simulink library "lib_Conduction_2DCondFullyImplicit"  (R2015a)
settings: Solver=ode45  StartTime=0.0  StopTime=10.0  RelTol=1e-3
libraries: lib_GenTools_SubMatrix x24
(part 2 of 2)

== matlab function lib_Conduction_2DCondFullyImplicit/2D Transient Conduction Model - Fully Implicit/MATLAB Function ==
  data: kx input; ky input; T output; Cp input; rho input; TfL input; hL input; TsL input; CL input; TrL input; uL input; TfR input; hR input; TsR input; CR input; TrR input; uR input; TfB input; hB input; TsB input; CB input; TrB input; uB input; TfT input; hT input; TsT input; CT input; TrT input; uT input; x input; y input; shape input; AL input; AR input; AB input; AT input; VL input; VR input; VB input; VT input; JLx input; JLy input; JRx input; JRy input; JBx input; JBy input; JTx input; JTy input; dt input; To input; Erro input; Err output; BN input
function [T,Err] = HeatX2DQuasi(kx,ky,Cp,rho,TfL,hL,...
    TsL,CL,TrL,uL,TfR,hR,TsR,CR,...
    TrR,uR,TfB,hB,TsB,CB,TrB,uB,TfT,hT,...
    TsT,CT,TrT,uT,x,y,shape,...
    AL,AR,AB,AT,VL,VR,VB,VT,JLx,JLy,JRx,JRy,...
    JBx,JBy,JTx,JTy,dt,To,Erro,BN)
%#codegen

% Written by: Jonathan Kratz, NASA GRC
% Date: January 27, 2017
%
% Description: This MATLAB function block solves a 2-D heat transfer
% problem with the potential for various boundary conditions including
% convection, conduction, and radiation. The function is capable of
% accepting time-varying thermal properties including the conductivity,
% specific heat, and density of the solid structure. Heat transfer
% coefficients can also be time-varying. The function is equiped to handle
% planar and cylindrical geometries. A generic non-uniform spatial
% discretization may be used but a constant time-step is encouraged for
% accuracy in time. The governing equation is below:
%                  _                                                  _
%   dT     1      |  /dk   a*k \ dT     d2T    /dk   q*k \  dT     d2T |
%   -- = ------ * | | -- + ---- |-- + k --- + | -- + ---- | -- + k --- |
%   dt   rho*Cp   |_ \dy    dy / dy     dy2    \dx    dx /  dx     dx2_|
%
% Generally the geometry will be planar in the x or y direction but could be
% axisymmetric (cylindrical) in the other direction. This equation is
% discretized and to form a system of linear equations and solved using a 2-D
% implicit scheme. The Crank-Nicolson Method is applied to the discretizied 
% equation and the linear algreba techniques are used to solve the system of 
% equations. The boundary conditions use linear heat transfer 
% coefficients and it is suggested that these coefficients be evaluated 
% using thermal properties of the previous time-step (i.e. temperature of 
% the structure and thermodynamic properties of the surrounding gases).
% Depending on the problem they may be assumed constant.
%
% Inputs:
%   Note m is the number of nodes in y-dir and n is the number of
%   nodes in the x-dir.
% Thermal Properties:
%   kx - thermal conductivity of the structure in x-dir [m x n]
%   ky - thermal conductivity of the structure in y-dir [m x n]
%   Cp - heat capacity of the structure [m x n]
%   rho - density of the structure [m x n]
% Boundary Conditions:
%   TfL - temperature of fluid on the left surface [m x 1]
%   hL - convective heat transfer coefficient on the left surface [m x 1]
%   CL - thermal conductance of contacting structure on the left surface 
%        [m x 1]
%   TsL - temperature of a contacting structure on the left surface [m x 1]
%   TrL - temperature of a distant external radiating source/sink [m x 1]
%       exposed to the left surface
%   uL - linear radiative heat transfer coefficient between the left
%       surface and external radiating source/sink it is exposed to [m x 1]
%   TfR - temperature of fluid on the right surface [m x 1]
%   hR - convective heat transfer coefficient on the right surface [m x 1]
%   TsR - temperature of a contacting structure on the right surface [m x 1]
%   CR - thermal conductance of contacting structure on the right surface 
%        [m x 1]
%   TrR - temperature of a distant external radiating source/sink
%       exposed to the right surface [m x 1]
%   uR - linear radiative heat transfer coefficient between the right
%       surface and external radiating source/sink it is exposed to [m x 1]
%   TfB - temperature of fluid on the bottom surface [n x 1]
%   hB - convective heat transfer coefficient on the bottom surface [n x 1]
%   TsB - temperature of a contacting structure on the bottom surface [n x 1]
%   CB - thermal conductance of contacting structure on the bottom surface 
%        [n x 1]
%   TrB - temperature of a distant external radiating source/sink 
%       exposed to the bottom surface [n x 1]
%   uB - linear radiative heat transfer coefficient between the bottom
%       surface and external radiating source/sink it is exposed to [n x 1]
%   TfT - temperature of fluid on the top surface [n x 1]
%   hT - convective heat transfer coefficient on the top surface [n x 1]
%   TsT - temperature of a contacting structure on the top surface [n x 1]
%   CT - thermal conductance of contacting structure on the top surface 
%        [n x 1]
%   TrT - temperature of a distant external radiating source/sink 
%       exposed to the top surface [n x 1]
%   uT - linear radiative heat transfer coefficient between the top
%       surface and external radiating source/sink it is exposed to [n x 1]
% Boundary Node Properties
%   AL - surface area of the left surface nodes [m x 1]
%   AR - surface area of the right surface nodes [m x 1]
%   AB - surface area of the bottom surface nodes [n x 1]
%   AT - surface area of the top surface nodes [n x 1]
%   VL - volume of the left surface nodes [m x 1]
%   VR - volume of the right surface nodes [m x 1]
%   VB - volume of the bottom surface nodes [n x 1]
%   VT - volume of the top surface nodes [n x 1]
%   JL - thermal resistance * k of the left surface nodes [m x 1]
%   JR - thermal resistance * k of the right surface nodes [m x 1]
%   JB - thermal resistance * k of the bottom surface nodes [n x 1]
%   JT - thermal resistance * k of the top surface nodes [n x 1]
% Geometry/Discretization:
%   x - discretized spatial coordinates in x-direction [n]
%   y - discretized spatial coordinates in r- or y-direction [m]
%   shape - shape parameter 
% Solver:
%   dt - time-step of the solver [1 x 1]
%   To - initial/previous condition for the solver/initial temperature of 
%       the structure [m x n]
% Error/Warning Detection
%   Erro - array with error states. Tracks errors/warnings that have been
%       detected. [number of error checks x 1]
%   BN - block name. Used in warning messages.
%
% Outputs:
%   T - Matrix of temperature at each node [m x n]
%   Err - array with updated error states. [number of error checks x 1]
%  
% Discretization guidelines: The first and last nodes should be on the 
% surface. It is important that that the first node should be half the size 
% as the second node and the last node should be half the size of the 
% second to last node. This is due to the assumptions made in the 
% formulization of the boundary condition equations. Also, for planar 
% geometries the first value of the discretization array x (which 
% corresponds to the first node) can be any real numeric value (it does not
% have to be zero, equations use node size so relative position is what 
% matters). In the case of a cylindrical geometry the first value in the x 
% array should be the inner radius of the structure. It should go without 
% saying that the spatial discretization array x is required to be 
% montonically increasing.

% shape factor
a = 0;
q = 0;
if shape == 1
    a = 0;
    q = 0;
elseif shape == 2
    a = 1;
    q = 0;
elseif shape == 3
    a = 0;
    q = 1;
end

% number of elements
n = length(x); %number of nodes in x-dir
m = length(y); %number of nodes in y-dir

% initialize error/warning array
Err = Erro;
ErrNum = 1; %Error index

%180 Error Checks
% check sizes and contents -----------------------------------------------%
% ---- x ---- %
% Not Empty?
if isempty(x) == 1 && Err(ErrNum) < 1
    Err(ErrNum) = 1;
    fprintf('Warning in %s: x_M is an empty array.\n',char(BN));
end
ErrNum = ErrNum + 1;
% 1-D Array?
if (length(size(x)) ~= 2 && min(size(x)) ~= 1) && Err(ErrNum) < 1
    Err(ErrNum) = 1;
    fprintf('Warning in %s: x_M must be a 1-D array.\n',char(BN));
end
ErrNum = ErrNum + 1;
% Length >= 4?
if length(x) < 4 && Err(ErrNum) < 1
    Err(ErrNum) = 1;
    fprintf('Warning in %s: x_M must have at least 4 elements.\n',char(BN));
end
ErrNum = ErrNum + 1;
% Real?
if min(isreal(x)) < 1 && Err(ErrNum) < 1
    Err(ErrNum) = 1;
    fprintf('Warning in %s: x_M must have all real elements.\n',char(BN));
end
ErrNum = ErrNum + 1;
% Finite?
if min(isfinite(x)) < 1 && Err(ErrNum) < 1
    Err(ErrNum) = 1;
    fprintf('Warning in %s: x_M must have all finite elements.\n',char(BN));
end
ErrNum = ErrNum + 1;
% Monotonically Increasing?
if min(diff(x)) <= 0 && Err(ErrNum) < 1
    Err(ErrNum) = 1;
    fprintf('Warning in %s: x_M must be monotonically increasing.\n',char(BN));
end
ErrNum = ErrNum + 1;
% ---- y ---- %
% Not Empty?
if isempty(y) == 1 && Err(ErrNum) < 1
    Err(ErrNum) = 1;
    fprintf('Warning in %s: y_M is an empty array.\n',char(BN));
end
ErrNum = ErrNum + 1;
% 1-D Array?
if (length(size(y)) ~= 2 && min(size(y)) ~= 1) && Err(ErrNum) < 1
    Err(ErrNum) = 1;
    fprintf('Warning in %s: y_M must be a 2-D array.\n',char(BN));
end
ErrNum = ErrNum + 1;
% Number of rows >= 4?
if length(y) < 4 && Err(ErrNum) < 1
    Err(ErrNum) = 1;
    fprintf('Warning in %s: y_M must have at least 4 rows.\n',char(BN));
end
ErrNum = ErrNum + 1;
% Real?
if min(isreal(y)) < 1 && Err(ErrNum) < 1
    Err(ErrNum) = 1;
    fprintf('Warning in %s: y_M must have all real elements.\n',char(BN));
end
ErrNum = ErrNum + 1;
% Finite?
if min(isfinite(y)) < 1 && Err(ErrNum) < 1
    Err(ErrNum) = 1;
    fprintf('Warning in %s: y_M must have all finite elements.\n',char(BN));
end
ErrNum = ErrNum + 1;
% y is Monotonically Increasing?
if min(diff(y)) <= 0 && Err(ErrNum) < 1
    Err(ErrNum) = 1;
    fprintf('Warning in %s: y_M must be monotonically increasing.\n',char(BN));
end
ErrNum = ErrNum + 1;
% ---- kx ---- %
% Not Empty?
if isempty(kx) == 1 && Err(ErrNum) < 1
    Err(ErrNum) = 1;
    fprintf('Warning in %s: kx is an empty array.\n',char(BN));
end
ErrNum = ErrNum + 1;
% Size of To?
if (size(kx,1) ~= m && size(kx,2) ~= n) && Err(ErrNum) < 1
    Err(ErrNum) = 1;
    fprintf('Warning in %s: kx must have as many rows a elements in y and as many columns a elements in x.\n',char(BN));
end
ErrNum = ErrNum + 1;
% Real?
if min(isreal(kx)) < 1 && Err(ErrNum) < 1
    Err(ErrNum) = 1;
    fprintf('Warning in %s: kx must have all real elements.\n',char(BN));
end
ErrNum = ErrNum + 1;
% Finite?
if min(min(isfinite(kx))) < 1 && Err(ErrNum) < 1
    Err(ErrNum) = 1;
    fprintf('Warning in %s: kx must have all finite elements.\n',char(BN));
end
ErrNum = ErrNum + 1;
% Positive?
if min(min(kx)) <= 0 && Err(ErrNum) < 1
    Err(ErrNum) = 1;
    fprintf('Warning in %s: kx must have all positive elements.\n',char(BN));
end
ErrNum = ErrNum + 1;
% ---- ky ---- %
% Not Empty?
if isempty(ky) == 1 && Err(ErrNum) < 1
    Err(ErrNum) = 1;
    fprintf('Warning in %s: ky is an empty array.\n',char(BN));
end
ErrNum = ErrNum + 1;
% Size of y?
if (size(ky,1) ~= m && size(ky,2) ~= n) && Err(ErrNum) < 1
    Err(ErrNum) = 1;
    fprintf('Warning in %s: ky must have as many rows as elements in y and as many columns as elements in x.\n',char(BN));
end
ErrNum = ErrNum + 1;
% Real?
if min(isreal(ky)) < 1 && Err(ErrNum) < 1
    Err(ErrNum) = 1;
    fprintf('Warning in %s: ky must have all real elements.\n',char(BN));
end
ErrNum = ErrNum + 1;
% Finite?
if min(min(isfinite(ky))) < 1 && Err(ErrNum) < 1
    Err(ErrNum) = 1;
    fprintf('Warning in %s: ky must have all finite elements.\n',char(BN));
end
ErrNum = ErrNum + 1;
% Positive?
if min(min(ky)) <= 0 && Err(ErrNum) < 1
    Err(ErrNum) = 1;
    fprintf('Warning in %s: ky must have all positive elements.\n',char(BN));
end
ErrNum = ErrNum + 1;
% ---- Cp ---- %
% Not Empty?
if isempty(Cp) == 1 && Err(ErrNum) < 1
    Err(ErrNum) = 1;
    fprintf('Warning in %s: Cp is an empty array.\n',char(BN));
end
ErrNum = ErrNum + 1;
% Size of y?
if (size(Cp,1) ~= m && size(Cp,2) ~= n) && Err(ErrNum) < 1
    Err(ErrNum) = 1;
    fprintf('Warning in %s: Cp must have as many rows as elements in y and as many columns as elements in x.\n',char(BN));
end
ErrNum = ErrNum + 1;
% Real?
if min(isreal(Cp)) < 1 && Err(ErrNum) < 1
    Err(ErrNum) = 1;
    fprintf('Warning in %s: Cp must have all real elements.\n',char(BN));
end
ErrNum = ErrNum + 1;
% Finite?
if min(min(isfinite(Cp))) < 1 && Err(ErrNum) < 1
    Err(ErrNum) = 1;
    fprintf('Warning in %s: Cp must have all finite elements.\n',char(BN));
end
ErrNum = ErrNum + 1;
% Positive?
if min(min(Cp)) <= 0 && Err(ErrNum) < 1
    Err(ErrNum) = 1;
    fprintf('Warning in %s: Cp must have all positive elements.\n',char(BN));
end
ErrNum = ErrNum + 1;
% ---- rho ---- %
% Not Empty?
if isempty(rho) == 1 && Err(ErrNum) < 1
    Err(ErrNum) = 1;
    fprintf('Warning in %s: rho is an empty array.\n',char(BN));
end
ErrNum = ErrNum + 1;
% Size of y?
if (size(rho,1) ~= m && size(rho,2) ~= n) && Err(ErrNum) < 1
    Err(ErrNum) = 1;
    fprintf('Warning in %s: rho must have as many rows as elements in y and as many columns as elements in x.\n',char(BN));
end
ErrNum = ErrNum + 1;
% Real?
if min(isreal(rho)) < 1 && Err(ErrNum) < 1
    Err(ErrNum) = 1;
    fprintf('Warning in %s: rho must have all real elements.\n',char(BN));
end
ErrNum = ErrNum + 1;
% Finite?
if min(min(isfinite(rho))) < 1 && Err(ErrNum) < 1
    Err(ErrNum) = 1;
    fprintf('Warning in %s: rho must have all finite elements.\n',char(BN));
end
ErrNum = ErrNum + 1;
% Positive?
if min(min(rho)) <= 0 && Err(ErrNum) < 1
    Err(ErrNum) = 1;
    fprintf('Warning in %s: rho must have all positive elements.\n',char(BN));
end
ErrNum = ErrNum + 1;
% ---- dt ---- %
% Scalar?
if isscalar(dt) < 1 && Err(ErrNum) < 1
    Err(ErrNum) = 1;
    fprintf('Warning in %s: dt_M must be a scalar.\n',char(BN));
end
ErrNum = ErrNum + 1;
% Real?
if isreal(dt) < 1 && Err(ErrNum) < 1
    Err(ErrNum) = 1;
    fprintf('Warning in %s: dt_M must be real.\n',char(BN));
end
ErrNum = ErrNum + 1;
% Finite?
if isfinite(dt) < 1 && Err(ErrNum) < 1
    Err(ErrNum) = 1;
    fprintf('Warning in %s: dt_M must be finite.\n',char(BN));
end
ErrNum = ErrNum + 1;
% Positive?
if dt <= 0 && Err(ErrNum) < 1
    Err(ErrNum) = 1;
    fprintf('Warning in %s: dt must be positive.\n',char(BN));
end
ErrNum = ErrNum + 1;
% ---- To ---- %
% Not Empty?
if isempty(To) == 1 && Err(ErrNum) < 1
    Err(ErrNum) = 1;
    fprintf('Warning in %s: To is an empty array.\n',char(BN));
end
ErrNum = ErrNum + 1;
% Size of y?
if (size(To,1) ~= m && size(To,2) ~= n) && Err(ErrNum) < 1
    Err(ErrNum) = 1;
    fprintf('Warning in %s: To must have as many rows as elements in y and as many columns as elements in x.\n',char(BN));
end
ErrNum = ErrNum + 1;
% Real?
if min(isreal(To)) < 1 && Err(ErrNum) < 1
    Err(ErrNum) = 1;
    fprintf('Warning in %s: To must have all real elements.\n',char(BN));
end
ErrNum = ErrNum + 1;
% Finite?
if min(min(isfinite(To))) < 1 && Err(ErrNum) < 1
    Err(ErrNum) = 1;
    fprintf('Warning in %s: To must have all finite elements.\n',char(BN));
end
ErrNum = ErrNum + 1;
% ---- TfL ---- %
% Not Empty?
if isempty(TfL) == 1 && Err(ErrNum) < 1
    Err(ErrNum) = 1;
    fprintf('Warning in %s: TfL is an empty array.\n',char(BN));
end
ErrNum = ErrNum + 1;
% 1-D Array?
if (min(size(TfL)) > 1 || length(size(TfL)) > 2) && Err(ErrNum) < 1
    Err(ErrNum) = 1;
    fprintf('Warning in %s: TfL must be a 1-D array.\n',char(BN));
end
ErrNum = ErrNum + 1;
% Length of number of elements in y?
if length(TfL) ~= length(y) && Err(ErrNum) < 1
    Err(ErrNum) = 1;
    fprintf('Warning in %s: TfL have as many elements as y.\n',char(BN));
end
ErrNum = ErrNum + 1;
% Real?
if min(isreal(TfL)) < 1 && Err(ErrNum) < 1
    Err(ErrNum) = 1;
    fprintf('Warning in %s: TfL must have all real elments.\n',char(BN));
end
ErrNum = ErrNum + 1;
% Finite?
if min(isfinite(TfL)) < 1 && Err(ErrNum) < 1
    Err(ErrNum) = 1;
    fprintf('Warning in %s: TfL must have all finite elements.\n',char(BN));
end
ErrNum = ErrNum + 1;
% ---- hL ---- %
% Not Empty?
if isempty(hL) == 1 && Err(ErrNum) < 1
    Err(ErrNum) = 1;
    fprintf('Warning in %s: hL is an empty array.\n',char(BN));
end
ErrNum = ErrNum + 1;
% 1-D Array?
if (min(size(hL)) > 1 || length(size(hL)) > 2) && Err(ErrNum) < 1
    Err(ErrNum) = 1;
    fprintf('Warning in %s: hL must be a 1-D array.\n',char(BN));
end
ErrNum = ErrNum + 1;
% Length of number of elements in y?
if length(hL) ~= length(y) && Err(ErrNum) < 1
    Err(ErrNum) = 1;
    fprintf('Warning in %s: hL have as many elements as y.\n',char(BN));
end
ErrNum = ErrNum + 1;
% Real?
if min(isreal(hL)) < 1 && Err(ErrNum) < 1
    Err(ErrNum) = 1;
    fprintf('Warning in %s: hL must have all real elments.\n',char(BN));
end
ErrNum = ErrNum + 1;
% Finite?
if min(isfinite(hL)) < 1 && Err(ErrNum) < 1
    Err(ErrNum) = 1;
    fprintf('Warning in %s: hL must have all finite elements.\n',char(BN));
end
ErrNum = ErrNum + 1;
% ---- TsL ---- %
% Not Empty?
if isempty(TsL) == 1 && Err(ErrNum) < 1
    Err(ErrNum) = 1;
    fprintf('Warning in %s: TsL is an empty array.\n',char(BN));
end
ErrNum = ErrNum + 1;
% 1-D Array?
if (min(size(TsL)) > 1 || length(size(TsL)) > 2) && Err(ErrNum) < 1
    Err(ErrNum) = 1;
    fprintf('Warning in %s: TsL must be a 1-D array.\n',char(BN));
end
ErrNum = ErrNum + 1;
% Length of number of elements in y?
if length(TsL) ~= length(y) && Err(ErrNum) < 1
    Err(ErrNum) = 1;
    fprintf('Warning in %s: TsL have as many elements as y.\n',char(BN));
end
ErrNum = ErrNum + 1;
% Real?
if min(isreal(TsL)) < 1 && Err(ErrNum) < 1
    Err(ErrNum) = 1;
    fprintf('Warning in %s: TsL must have all real elments.\n',char(BN));
end
ErrNum = ErrNum + 1;
% Finite?
if min(isfinite(TsL)) < 1 && Err(ErrNum) < 1
    Err(ErrNum) = 1;
    fprintf('Warning in %s: TsL must have all finite elements.\n',char(BN));
end
ErrNum = ErrNum + 1;
% ---- CL ---- %
% Not Empty?
if isempty(CL) == 1 && Err(ErrNum) < 1
    Err(ErrNum) = 1;
    fprintf('Warning in %s: CL is an empty array.\n',char(BN));
end
ErrNum = ErrNum + 1;
% 1-D Array?
if (min(size(CL)) > 1 || length(size(CL)) > 2) && Err(ErrNum) < 1
    Err(ErrNum) = 1;
    fprintf('Warning in %s: CL must be a 1-D array.\n',char(BN));
end
ErrNum = ErrNum + 1;
% Length of number of elements in y?
if length(CL) ~= length(y) && Err(ErrNum) < 1
    Err(ErrNum) = 1;
    fprintf('Warning in %s: CL have as many elements as y.\n',char(BN));
end
ErrNum = ErrNum + 1;
% Real?
if min(isreal(CL)) < 1 && Err(ErrNum) < 1
    Err(ErrNum) = 1;
    fprintf('Warning in %s: CL must have all real elments.\n',char(BN));
end
ErrNum = ErrNum + 1;
% Finite?
if min(isfinite(CL)) < 1 && Err(ErrNum) < 1
    Err(ErrNum) = 1;
    fprintf('Warning in %s: CL must have all finite elements.\n',char(BN));
end
ErrNum = ErrNum + 1;
% ---- TrL ---- %
% Not Empty?
if isempty(TrL) == 1 && Err(ErrNum) < 1
    Err(ErrNum) = 1;
    fprintf('Warning in %s: TrL is an empty array.\n',char(BN));
end
ErrNum = ErrNum + 1;
% 1-D Array?
if (min(size(TrL)) > 1 || length(size(TrL)) > 2) && Err(ErrNum) < 1
    Err(ErrNum) = 1;
    fprintf('Warning in %s: TrL must be a 1-D array.\n',char(BN));
end
ErrNum = ErrNum + 1;
% Length of number of elements in y?
if length(TrL) ~= length(y) && Err(ErrNum) < 1
    Err(ErrNum) = 1;
    fprintf('Warning in %s: TrL have as many elements as y.\n',char(BN));
end
ErrNum = ErrNum + 1;
% Real?
if min(isreal(TrL)) < 1 && Err(ErrNum) < 1
    Err(ErrNum) = 1;
    fprintf('Warning in %s: TrL must have all real elments.\n',char(BN));
end
ErrNum = ErrNum + 1;
% Finite?
if min(isfinite(TrL)) < 1 && Err(ErrNum) < 1
    Err(ErrNum) = 1;
    fprintf('Warning in %s: TrL must have all finite elements.\n',char(BN));
end
ErrNum = ErrNum + 1;
% ---- uL ---- %
% Not Empty?
if isempty(uL) == 1 && Err(ErrNum) < 1
    Err(ErrNum) = 1;
    fprintf('Warning in %s: uL is an empty array.\n',char(BN));
end
ErrNum = ErrNum + 1;
% 1-D Array?
if (min(size(uL)) > 1 || length(size(uL)) > 2) && Err(ErrNum) < 1
    Err(ErrNum) = 1;
    fprintf('Warning in %s: uL must be a 1-D array.\n',char(BN));
end
ErrNum = ErrNum + 1;
% Length of number of elements in y?
if length(uL) ~= length(y) && Err(ErrNum) < 1
    Err(ErrNum) = 1;
    fprintf('Warning in %s: uL have as many elements as y.\n',char(BN));
end
ErrNum = ErrNum + 1;
% Real?
if min(isreal(uL)) < 1 && Err(ErrNum) < 1
    Err(ErrNum) = 1;
    fprintf('Warning in %s: uL must have all real elments.\n',char(BN));
end
ErrNum = ErrNum + 1;
% Finite?
if min(isfinite(uL)) < 1 && Err(ErrNum) < 1
    Err(ErrNum) = 1;
    fprintf('Warning in %s: uL must have all finite elements.\n',char(BN));
end
ErrNum = ErrNum + 1;
% ---- TfR ---- %
% Not Empty?
if isempty(TfR) == 1 && Err(ErrNum) < 1
    Err(ErrNum) = 1;
    fprintf('Warning in %s: TfR is an empty array.\n',char(BN));
end
ErrNum = ErrNum + 1;
% 1-D Array?
if (min(size(TfR)) > 1 || length(size(TfR)) > 2) && Err(ErrNum) < 1
    Err(ErrNum) = 1;
    fprintf('Warning in %s: TfR must be a 1-D array.\n',char(BN));
end
ErrNum = ErrNum + 1;
% Length of number of elements in y?
if length(TfR) ~= length(y) && Err(ErrNum) < 1
    Err(ErrNum) = 1;
    fprintf('Warning in %s: TfR have as many elements as y.\n',char(BN));
end
ErrNum = ErrNum + 1;
% Real?
if min(isreal(TfR)) < 1 && Err(ErrNum) < 1
    Err(ErrNum) = 1;
    fprintf('Warning in %s: TfR must have all real elments.\n',char(BN));
end
ErrNum = ErrNum + 1;
% Finite?
if min(isfinite(TfR)) < 1 && Err(ErrNum) < 1
    Err(ErrNum) = 1;
    fprintf('Warning in %s: TfR must have all finite elements.\n',char(BN));
end
ErrNum = ErrNum + 1;
% ---- hR ---- %
% Not Empty?
if isempty(hR) == 1 && Err(ErrNum) < 1
    Err(ErrNum) = 1;
    fprintf('Warning in %s: hR is an empty array.\n',char(BN));
end
ErrNum = ErrNum + 1;
% 1-D Array?
if (min(size(hR)) > 1 || length(size(hR)) > 2) && Err(ErrNum) < 1
    Err(ErrNum) = 1;
    fprintf('Warning in %s: hR must be a 1-D array.\n',char(BN));
end
ErrNum = ErrNum + 1;
% Length of number of elements in y?
if length(hR) ~= length(y) && Err(ErrNum) < 1
    Err(ErrNum) = 1;
    fprintf('Warning in %s: hR have as many elements as y.\n',char(BN));
end
ErrNum = ErrNum + 1;
% Real?
if min(isreal(hR)) < 1 && Err(ErrNum) < 1
    Err(ErrNum) = 1;
    fprintf('Warning in %s: hR must have all real elments.\n',char(BN));
end
ErrNum = ErrNum + 1;
% Finite?
if min(isfinite(hR)) < 1 && Err(ErrNum) < 1
    Err(ErrNum) = 1;
    fprintf('Warning in %s: hR must have all finite elements.\n',char(BN));
end
ErrNum = ErrNum + 1;
% ---- TsR ---- %
% Not Empty?
if isempty(TsR) == 1 && Err(ErrNum) < 1
    Err(ErrNum) = 1;
    fprintf('Warning in %s: TsR is an empty array.\n',char(BN));
end
ErrNum = ErrNum + 1;
% 1-D Array?
if (min(size(TsR)) > 1 || length(size(TsR)) > 2) && Err(ErrNum) < 1
    Err(ErrNum) = 1;
    fprintf('Warning in %s: TsR must be a 1-D array.\n',char(BN));
end
ErrNum = ErrNum + 1;
% Length of number of elements in y?
if length(TsR) ~= length(y) && Err(ErrNum) < 1
    Err(ErrNum) = 1;
    fprintf('Warning in %s: TsR have as many elements as y.\n',char(BN));
end
ErrNum = ErrNum + 1;
% Real?
if min(isreal(TsR)) < 1 && Err(ErrNum) < 1
    Err(ErrNum) = 1;
    fprintf('Warning in %s: TsR must have all real elments.\n',char(BN));
end
ErrNum = ErrNum + 1;
% Finite?
if min(isfinite(TsR)) < 1 && Err(ErrNum) < 1
    Err(ErrNum) = 1;
    fprintf('Warning in %s: TsR must have all finite elements.\n',char(BN));
end
ErrNum = ErrNum + 1;
% ---- CR ---- %
% Not Empty?
if isempty(CR) == 1 && Err(ErrNum) < 1
    Err(ErrNum) = 1;
    fprintf('Warning in %s: CR is an empty array.\n',char(BN));
end
ErrNum = ErrNum + 1;
% 1-D Array?
if (min(size(CR)) > 1 || length(size(CR)) > 2) && Err(ErrNum) < 1
    Err(ErrNum) = 1;
    fprintf('Warning in %s: CR must be a 1-D array.\n',char(BN));
end
ErrNum = ErrNum + 1;
% Length of number of elements in y?
if length(CR) ~= length(y) && Err(ErrNum) < 1
    Err(ErrNum) = 1;
    fprintf('Warning in %s: CR have as many elements as y.\n',char(BN));
end
ErrNum = ErrNum + 1;
% Real?
if min(isreal(CR)) < 1 && Err(ErrNum) < 1
    Err(ErrNum) = 1;
    fprintf('Warning in %s: CR must have all real elments.\n',char(BN));
end
ErrNum = ErrNum + 1;
% Finite?
if min(isfinite(CR)) < 1 && Err(ErrNum) < 1
    Err(ErrNum) = 1;
    fprintf('Warning in %s: CR must have all finite elements.\n',char(BN));
end
ErrNum = ErrNum + 1;
% ---- TrR ---- %
% Not Empty?
if isempty(TrR) == 1 && Err(ErrNum) < 1
    Err(ErrNum) = 1;
    fprintf('Warning in %s: TrR is an empty array.\n',char(BN));
end
ErrNum = ErrNum + 1;
% 1-D Array?
if (min(size(TrR)) > 1 || length(size(TrR)) > 2) && Err(ErrNum) < 1
    Err(ErrNum) = 1;
    fprintf('Warning in %s: TrR must be a 1-D array.\n',char(BN));
end
ErrNum = ErrNum + 1;
% Length of number of elements in y?
if length(TrR) ~= length(y) && Err(ErrNum) < 1
    Err(ErrNum) = 1;
    fprintf('Warning in %s: TrR have as many elements as y.\n',char(BN));
end
ErrNum = ErrNum + 1;
% Real?
if min(isreal(TrR)) < 1 && Err(ErrNum) < 1
    Err(ErrNum) = 1;
    fprintf('Warning in %s: TrR must have all real elments.\n',char(BN));
end
ErrNum = ErrNum + 1;
% Finite?
if min(isfinite(TrR)) < 1 && Err(ErrNum) < 1
    Err(ErrNum) = 1;
    fprintf('Warning in %s: TrR must have all finite elements.\n',char(BN));
end
ErrNum = ErrNum + 1;
% ---- uR ---- %
% Not Empty?
if isempty(uR) == 1 && Err(ErrNum) < 1
    Err(ErrNum) = 1;
    fprintf('Warning in %s: uR is an empty array.\n',char(BN));
end
ErrNum = ErrNum + 1;
% 1-D Array?
if (min(size(uR)) > 1 || length(size(uR)) > 2) && Err(ErrNum) < 1
    Err(ErrNum) = 1;
    fprintf('Warning in %s: uR must be a 1-D array.\n',char(BN));
end
ErrNum = ErrNum + 1;
% Length of number of elements in y?
if length(uR) ~= length(y) && Err(ErrNum) < 1
    Err(ErrNum) = 1;
    fprintf('Warning in %s: uR have as many elements as y.\n',char(BN));
end
ErrNum = ErrNum + 1;
% Real?
if min(isreal(uR)) < 1 && Err(ErrNum) < 1
    Err(ErrNum) = 1;
    fprintf('Warning in %s: uR must have all real elments.\n',char(BN));
end
ErrNum = ErrNum + 1;
% Finite?
if min(isfinite(uR)) < 1 && Err(ErrNum) < 1
    Err(ErrNum) = 1;
    fprintf('Warning in %s: uR must have all finite elements.\n',char(BN));
end
ErrNum = ErrNum + 1;
% ---- TfB ---- %
% Not Empty?
if isempty(TfB) == 1 && Err(ErrNum) < 1
    Err(ErrNum) = 1;
    fprintf('Warning in %s: TfB is an empty array.\n',char(BN));
end
ErrNum = ErrNum + 1;
% 1-D Array?
if (min(size(TfB)) > 1 || length(size(TfB)) > 2) && Err(ErrNum) < 1
    Err(ErrNum) = 1;
    fprintf('Warning in %s: TfB must be a 1-D array.\n',char(BN));
end
ErrNum = ErrNum + 1;
% Length of x?
if length(TfB) ~= length(x) && Err(ErrNum) < 1
    Err(ErrNum) = 1;
    fprintf('Warning in %s: TfB must have as many elements as x.\n',char(BN));
end
ErrNum = ErrNum + 1;
% Real?
if min(isreal(TfB)) < 1 && Err(ErrNum) < 1
    Err(ErrNum) = 1;
    fprintf('Warning in %s: TfB must have all real elments.\n',char(BN));
end
ErrNum = ErrNum + 1;
% Finite?
if min(isfinite(TfB)) < 1 && Err(ErrNum) < 1
    Err(ErrNum) = 1;
    fprintf('Warning in %s: TfB must have all finite elements.\n',char(BN));
end
ErrNum = ErrNum + 1;
% ---- hB ---- %
% Not Empty?
if isempty(hB) == 1 && Err(ErrNum) < 1
    Err(ErrNum) = 1;
    fprintf('Warning in %s: hB is an empty array.\n',char(BN));
end
ErrNum = ErrNum + 1;
% 1-D Array?
if (min(size(hB)) > 1 || length(size(hB)) > 2) && Err(ErrNum) < 1
    Err(ErrNum) = 1;
    fprintf('Warning in %s: hB must be a 1-D array.\n',char(BN));
end
ErrNum = ErrNum + 1;
% Length of x?
if length(hB) ~= length(x) && Err(ErrNum) < 1
    Err(ErrNum) = 1;
    fprintf('Warning in %s: hB have as many elements as x.\n',char(BN));
end
ErrNum = ErrNum + 1;
% Real?
if min(isreal(hB)) < 1 && Err(ErrNum) < 1
    Err(ErrNum) = 1;
    fprintf('Warning in %s: hB must have all real elments.\n',char(BN));
end
ErrNum = ErrNum + 1;
% Finite?
if min(isfinite(hB)) < 1 && Err(ErrNum) < 1
    Err(ErrNum) = 1;
    fprintf('Warning in %s: hB must have all finite elements.\n',char(BN));
end
ErrNum = ErrNum + 1;
% ---- TsB ---- %
% Not Empty?
if isempty(TsB) == 1 && Err(ErrNum) < 1
    Err(ErrNum) = 1;
    fprintf('Warning in %s: TsB is an empty array.\n',char(BN));
end
ErrNum = ErrNum + 1;
% 1-D Array?
if (min(size(TsB)) > 1 || length(size(TsB)) > 2) && Err(ErrNum) < 1
    Err(ErrNum) = 1;
    fprintf('Warning in %s: TsB must be a 1-D array.\n',char(BN));
end
ErrNum = ErrNum + 1;
% Length of x?
if length(TsB) ~= length(x) && Err(ErrNum) < 1
    Err(ErrNum) = 1;
    fprintf('Warning in %s: TsB have as many elements as x.\n',char(BN));
end
ErrNum = ErrNum + 1;
% Real?100
if min(isreal(TsB)) < 1 && Err(ErrNum) < 1
    Err(ErrNum) = 1;
    fprintf('Warning in %s: TsB must have all real elments.\n',char(BN));
end
ErrNum = ErrNum + 1;
% Finite?
if min(isfinite(TsB)) < 1 && Err(ErrNum) < 1
    Err(ErrNum) = 1;
    fprintf('Warning in %s: TsB must have all finite elements.\n',char(BN));
end
ErrNum = ErrNum + 1;
% ---- CB ---- %
% Not Empty?
if isempty(CB) == 1 && Err(ErrNum) < 1
    Err(ErrNum) = 1;
    fprintf('Warning in %s: CB is an empty array.\n',char(BN));
end
ErrNum = ErrNum + 1;
% 1-D Array?
if (min(size(CB)) > 1 || length(size(CB)) > 2) && Err(ErrNum) < 1
    Err(ErrNum) = 1;
    fprintf('Warning in %s: CB must be a 1-D array.\n',char(BN));
end
ErrNum = ErrNum + 1;
% Length of number of elements in x?
if length(CB) ~= length(x) && Err(ErrNum) < 1
    Err(ErrNum) = 1;
    fprintf('Warning in %s: CB must have as many elements as x.\n',char(BN));
end
ErrNum = ErrNum + 1;
% Real?
if min(isreal(CB)) < 1 && Err(ErrNum) < 1
    Err(ErrNum) = 1;
    fprintf('Warning in %s: CB must have all real elments.\n',char(BN));
end
ErrNum = ErrNum + 1;
% Finite?
if min(isfinite(CB)) < 1 && Err(ErrNum) < 1
    Err(ErrNum) = 1;
    fprintf('Warning in %s: CB must have all finite elements.\n',char(BN));
end
ErrNum = ErrNum + 1;
% ---- TrB ---- %
% Not Empty?
if isempty(TrB) == 1 && Err(ErrNum) < 1
    Err(ErrNum) = 1;
    fprintf('Warning in %s: TrB is an empty array.\n',char(BN));
end
ErrNum = ErrNum + 1;
% 1-D Array?
if (min(size(TrB)) > 1 || length(size(TrB)) > 2) && Err(ErrNum) < 1
    Err(ErrNum) = 1;
    fprintf('Warning in %s: TrB must be a 1-D array.\n',char(BN));
end
ErrNum = ErrNum + 1;
% Length of x?
if length(TrB) ~= length(x) && Err(ErrNum) < 1
    Err(ErrNum) = 1;
    fprintf('Warning in %s: TrB have as many elements as x.\n',char(BN));
end
ErrNum = ErrNum + 1;
% Real?
if min(isreal(TrB)) < 1 && Err(ErrNum) < 1
    Err(ErrNum) = 1;
    fprintf('Warning in %s: TrB must have all real elments.\n',char(BN));
end
ErrNum = ErrNum + 1;
% Finite?
if min(isfinite(TrB)) < 1 && Err(ErrNum) < 1
    Err(ErrNum) = 1;
    fprintf('Warning in %s: TrB must have all finite elements.\n',char(BN));
end
ErrNum = ErrNum + 1;
% ---- uB ---- %
% Not Empty?
if isempty(uB) == 1 && Err(ErrNum) < 1
    Err(ErrNum) = 1;
    fprintf('Warning in %s: uB is an empty array.\n',char(BN));
end
ErrNum = ErrNum + 1;
% 1-D Array?
if (min(size(uB)) > 1 || length(size(uB)) > 2) && Err(ErrNum) < 1
    Err(ErrNum) = 1;
    fprintf('Warning in %s: uB must be a 1-D array.\n',char(BN));
end
ErrNum = ErrNum + 1;
% Length of x?
if length(uB) ~= length(x) && Err(ErrNum) < 1
    Err(ErrNum) = 1;
    fprintf('Warning in %s: uB have as many elements as x.\n',char(BN));
end
ErrNum = ErrNum + 1;
% Real?
if min(isreal(uB)) < 1 && Err(ErrNum) < 1
    Err(ErrNum) = 1;
    fprintf('Warning in %s: uB must have all real elments.\n',char(BN));
end
ErrNum = ErrNum + 1;
% Finite?
if min(isfinite(uB)) < 1 && Err(ErrNum) < 1
    Err(ErrNum) = 1;
    fprintf('Warning in %s: uB must have all finite elements.\n',char(BN));
end
ErrNum = ErrNum + 1;
% ---- TfT ---- %
% Not Empty?
if isempty(TfT) == 1 && Err(ErrNum) < 1
    Err(ErrNum) = 1;
    fprintf('Warning in %s: TfT is an empty array.\n',char(BN));
end
ErrNum = ErrNum + 1;
% 1-D Array?
if (min(size(TfT)) > 1 || length(size(TfT)) > 2) && Err(ErrNum) < 1
    Err(ErrNum) = 1;
    fprintf('Warning in %s: TfT must be a 1-D array.\n',char(BN));
end
ErrNum = ErrNum + 1;
% Length of x?
if length(TfT) ~= length(x) && Err(ErrNum) < 1
    Err(ErrNum) = 1;
    fprintf('Warning in %s: TfT have as many elements as x.\n',char(BN));
end
ErrNum = ErrNum + 1;
% Real?
if min(isreal(TfT)) < 1 && Err(ErrNum) < 1
    Err(ErrNum) = 1;
    fprintf('Warning in %s: TfT must have all real elments.\n',char(BN));
end
ErrNum = ErrNum + 1;
% Finite?
if min(isfinite(TfT)) < 1 && Err(ErrNum) < 1
    Err(ErrNum) = 1;
    fprintf('Warning in %s: TfT must have all finite elements.\n',char(BN));
end
ErrNum = ErrNum + 1;
% ---- hT ---- %
% Not Empty?
if isempty(hT) == 1 && Err(ErrNum) < 1
    Err(ErrNum) = 1;
    fprintf('Warning in %s: hT is an empty array.\n',char(BN));
end
ErrNum = ErrNum + 1;
% 1-D Array?
if (min(size(hT)) > 1 || length(size(hT)) > 2) && Err(ErrNum) < 1
    Err(ErrNum) = 1;
    fprintf('Warning in %s: hT must be a 1-D array.\n',char(BN));
end
ErrNum = ErrNum + 1;
% Length of x?
if length(hT) ~= length(x) && Err(ErrNum) < 1
    Err(ErrNum) = 1;
    fprintf('Warning in %s: hT have as many elements as x.\n',char(BN));
end
ErrNum = ErrNum + 1;
% Real?
if min(isreal(hT)) < 1 && Err(ErrNum) < 1
    Err(ErrNum) = 1;
    fprintf('Warning in %s: hT must have all real elments.\n',char(BN));
end
ErrNum = ErrNum + 1;
% Finite?
if min(isfinite(hT)) < 1 && Err(ErrNum) < 1
    Err(ErrNum) = 1;
    fprintf('Warning in %s: hT must have all finite elements.\n',char(BN));
end
ErrNum = ErrNum + 1;
% ---- TsT ---- %
% Not Empty?
if isempty(TsT) == 1 && Err(ErrNum) < 1
    Err(ErrNum) = 1;
    fprintf('Warning in %s: TsT is an empty array.\n',char(BN));
end
ErrNum = ErrNum + 1;
% 1-D Array?
if (min(size(TsT)) > 1 || length(size(TsT)) > 2) && Err(ErrNum) < 1
    Err(ErrNum) = 1;
    fprintf('Warning in %s: TsT must be a 1-D array.\n',char(BN));
end
ErrNum = ErrNum + 1;
% Length of x?
if length(TsT) ~= length(x) && Err(ErrNum) < 1
    Err(ErrNum) = 1;
    fprintf('Warning in %s: TsT have as many elements as x has rows.\n',char(BN));
end
ErrNum = ErrNum + 1;
% Real?
if min(isreal(TsT)) < 1 && Err(ErrNum) < 1
    Err(ErrNum) = 1;
    fprintf('Warning in %s: TsT must have all real elments.\n',char(BN));
end
ErrNum = ErrNum + 1;
% Finite?
if min(isfinite(TsT)) < 1 && Err(ErrNum) < 1
    Err(ErrNum) = 1;
    fprintf('Warning in %s: TsT must have all finite elements.\n',char(BN));
end
ErrNum = ErrNum + 1;
% ---- CT ---- %
% Not Empty?
if isempty(CT) == 1 && Err(ErrNum) < 1
    Err(ErrNum) = 1;
    fprintf('Warning in %s: CT is an empty array.\n',char(BN));
end
ErrNum = ErrNum + 1;
% 1-D Array?
if (min(size(CT)) > 1 || length(size(CT)) > 2) && Err(ErrNum) < 1
    Err(ErrNum) = 1;
    fprintf('Warning in %s: CT must be a 1-D array.\n',char(BN));
end
ErrNum = ErrNum + 1;
% Length of number of elements in x?
if length(CT) ~= length(x) && Err(ErrNum) < 1
    Err(ErrNum) = 1;
    fprintf('Warning in %s: CT must have as many elements as x.\n',char(BN));
end
ErrNum = ErrNum + 1;
% Real?
if min(isreal(CT)) < 1 && Err(ErrNum) < 1
    Err(ErrNum) = 1;
    fprintf('Warning in %s: CT must have all real elments.\n',char(BN));
end
ErrNum = ErrNum + 1;
% Finite?
if min(isfinite(CT)) < 1 && Err(ErrNum) < 1
    Err(ErrNum) = 1;
    fprintf('Warning in %s: CT must have all finite elements.\n',char(BN));
end
ErrNum = ErrNum + 1;
% ---- TrT ---- %
% Not Empty?
if isempty(TrT) == 1 && Err(ErrNum) < 1
    Err(ErrNum) = 1;
    fprintf('Warning in %s: TrT is an empty array.\n',char(BN));
end
ErrNum = ErrNum + 1;
% 1-D Array?
if (min(size(TrT)) > 1 || length(size(TrT)) > 2) && Err(ErrNum) < 1
    Err(ErrNum) = 1;
    fprintf('Warning in %s: TrT must be a 1-D array.\n',char(BN));
end
ErrNum = ErrNum + 1;
% Length of x?
if length(TrT) ~= length(x) && Err(ErrNum) < 1
    Err(ErrNum) = 1;
    fprintf('Warning in %s: TrT have as many elements as x.\n',char(BN));
end
ErrNum = ErrNum + 1;
% Real?
if min(isreal(TrT)) < 1 && Err(ErrNum) < 1
    Err(ErrNum) = 1;
    fprintf('Warning in %s: TrT must have all real elments.\n',char(BN));
end
ErrNum = ErrNum + 1;
% Finite?
if min(isfinite(TrT)) < 1 && Err(ErrNum) < 1
    Err(ErrNum) = 1;
    fprintf('Warning in %s: TrT must have all finite elements.\n',char(BN));
end
ErrNum = ErrNum + 1;
% ---- uT ---- %
% Not Empty?
if isempty(uT) == 1 && Err(ErrNum) < 1
    Err(ErrNum) = 1;
    fprintf('Warning in %s: uT is an empty array.\n',char(BN));
end
ErrNum = ErrNum + 1;
% 1-D Array?
if (min(size(uT)) > 1 || length(size(uT)) > 2) && Err(ErrNum) < 1
    Err(ErrNum) = 1;
    fprintf('Warning in %s: uT must be a 1-D array.\n',char(BN));
end
ErrNum = ErrNum + 1;
% Length of x?
if length(uT) ~= length(x) && Err(ErrNum) < 1
    Err(ErrNum) = 1;
    fprintf('Warning in %s: uT have as many elements as x.\n',char(BN));
end
ErrNum = ErrNum + 1;
% Real?
if min(isreal(uT)) < 1 && Err(ErrNum) < 1
    Err(ErrNum) = 1;
    fprintf('Warning in %s: uT must have all real elments.\n',char(BN));
end
ErrNum = ErrNum + 1;
% Finite?
if min(isfinite(uT)) < 1 && Err(ErrNum) < 1
    Err(ErrNum) = 1;
    fprintf('Warning in %s: uT must have all finite elements.\n',char(BN));
end

% Build A matrix and b vector --------------------------------------------%

% Tvec = A\z
%   x = [T(1,1) T(1,2) ... T(1,n) T(2,1) T(2,2) ... T(2,n) ... T(m,1) T(m,2) ... T(m,n)]'
%        _                                                                            _
%   A = | (1+B1)   F1     0      .      .      0      C1     0      .      .      0    |
%       |   D1   (1+B2)   F2     0      .      .      0      C2     0      .      .    |
%       |   0      D2   (1+B3)   F3     0      .      .      0      .      0      .    |
%       |   .      0      D3     .      .      0      .      .      0      .      0    |
%       |   .      .      0      .      .      .      0      .      .      0      CN   |
%       |   0      .      .      0      .      .      .      0      .      .      0    | 
%       |   G1     0      .      .      0      .      .      .      0      .      .    | 
%       |   0      G2     0      .      .      0      .      .     FNm2    0      .    | 
%       |   .      0      .      0      .      .      0     DNm2 (1+BNm2) FNm1    0    |
%       |   .      .      0      .      0      .      .      0     DNm1 (1+BNm1)  FN   |
%       |_  0      .      .      0      GN     0      .      .      0     DN    (1+BN)_|
%   z = [z1 z2 ... zN]
% Steps:
%   (1) Construct the vectors B, C, D, F, G, z
%       Sizes - B: [(n*m) x 1]
%               D: [((n*m)-1) x 1]
%               F: [((n*m)-1) x 1]
%               C: [((n-1)*m) x 1]
%               G: [((n-1)*m) x 1]
%   (2) Build the A matrix from B, C, D, F, and G
%               A: [(n*m) x (n*m)]

% Initialize A matrix and vectors
A = zeros(n*m,n*m);
B = zeros(n*m,1);
D = zeros(n*m-1,1);
F = zeros(n*m-1,1);
C = zeros((m-1)*n,1);
G = zeros((m-1)*n,1);
z = zeros(n*m,1);

% Index Counters
indB = 1;
indD = 1;
indF = 1;
indC = 1;
indG = 1;
indz = 1;

% Time-step (adapted code for ADI scheme that used DT = dt/2 - rather than
% change every occurance of DT in the code the value is simply re-assigned
% to dt vs. dt/2)
DT = dt;

% Build vectors (B, C, D, F, G, z) ---------------------------------------%

% For each row of nodes (bottom to top)
for i = 1:m
    
    %For each node in the row (left to right)
    for j = 1:n
        
        %BOTTOM SURFACE
        if i == 1
            
            %BOTTOM LEFT CORNER NODE
            if j == 1
                
                %Fourier and Biot Numbers, etc.
                %left vars
                FoL = 0;
                BiL = hL(i)*AL(i)*JLx(i)/kx(i,j); %Boit number
                BiRadL = uL(i)*AL(i)*JLx(i)/kx(i,j); %analogous Boit number for radiation
                FosL = DT*CL(i)/(rho(i,j)*Cp(i,j)*VL(i));
                %right vars 
                FoR = DT*kx(i,j)*(1/JLx(i))/(rho(i,j)*Cp(i,j)*VL(i)); %Fourier number;
                BiR = 0;
                BiRadR = 0;
                FosR = 0;
                %bottom vars
                FoB = 0;
                BiB = hB(j)*AB(j)*JBy(j)/ky(i,j); %Boit number
                BiRadB = uB(j)*AB(j)*JBy(j)/ky(i,j); %analogous Boit number for radiation
                FosB = DT*CB(j)/(rho(i,j)*Cp(i,j)*VB(j));
                %top vars
                FoT = DT*ky(i,j)*(1/JBy(j))/(rho(i,j)*Cp(i,j)*VB(j)); %Fourier number;
                BiT = 0;
                BiRadT = 0;
                FosT = 0;
                
                %adjust Fourier numbers for material transiton
                delT = y(i+1) - y(i);
                delR = x(j+1) - x(j);
                % -- FoT ---------------------
                if (ky(i+1,j)/ky(i,j)) > 1.1 || (ky(i+1,j)/ky(i,j)) < 0.9 %detect change in material
                    FoT = (ky(i,j)*(delT/2)+ky(i+1,j)*(delT/2))*DT/(rho(i,j)*Cp(i,j)*delT*delT*delT);
                end
                % -- FoR -------------------------
                if (kx(i,j+1)/kx(i,j)) > 1.1 || (kx(i,j+1)/kx(i,j)) < 0.9 %detect change in material
                    FoR = (kx(i,j)*(delR/2)+kx(i,j+1)*(delR/2))*DT/(rho(i,j)*Cp(i,j)*delR*delR*delR);
                end
                
                %simplification variables
                b = 0.5*FoB + 0.5*FoT*BiB + 0.5*FoT*BiRadB + 0.5*FosB ...
                  + 0.5*FoT + 0.5*FoB*BiT + 0.5*FoB*BiRadT + 0.5*FosT ...
                  + 0.5*FoL + 0.5*FoR*BiL + 0.5*FoR*BiRadL + 0.5*FosL ...
                  + 0.5*FoR + 0.5*FoL*BiR + 0.5*FoL*BiRadR + 0.5*FosR;
                c = -0.5*FoT;
                f = -0.5*FoR;
                BCs = FosB*TsB(j) + FoT*BiB*TfB(j) + FoT*BiRadB*TrB(j) ...
                    + FosL*TsL(i) + FoR*BiL*TfL(i) + FoR*BiRadL*TrL(i);
                
                %assign vector values
                B(indB) = 1+b;
                C(indC) = c;
                F(indF) = f;
                z(indz) = (1-b)*To(i,j) - c*To(i+1,j) - f*To(i,j+1) + BCs;
                
                %update indices
                indB = indB + 1;
                indC = indC + 1;
                indF = indF + 1;
                indz = indz + 1;
   
            %BOTTOM RIGHT CORNER NODE
            elseif j == n
                
                %Fourier and Biot Numbers
                %left vars
                FoL = DT*kx(i,j)*(1/JRx(i))/(rho(i,j)*Cp(i,j)*VR(i)); %Fourier number;
                BiL = 0;
                BiRadL = 0;
                FosL = 0;
                %right vars (conduction)
                FoR = 0;
                BiR = hR(i)*AR(i)*JRx(i)/kx(i,j); %Boit number
                BiRadR = uR(i)*AR(i)*JRx(i)/kx(i,j); %analogous Boit number for radiation
                FosR = DT*CR(i)/(rho(i,j)*Cp(i,j)*VR(i));
                %bottom vars
                FoB = 0;
                BiB = hB(j)*AB(j)*JBy(j)/ky(i,j); %Boit number
                BiRadB = uB(j)*AB(j)*JBy(j)/ky(i,j); %analogous Boit number for radiation
                FosB = DT*CB(j)/(rho(i,j)*Cp(i,j)*VB(j));
                %top vars
                FoT = DT*ky(i,j)*(1/JBy(j))/(rho(i,j)*Cp(i,j)*VB(j)); %Fourier number;
                BiT = 0;
                BiRadT = 0;
                FosT = 0;
                
                %adjust Fourier numbers for material transiton
                delT = y(i+1) - y(i);
                delL = x(j) - x(j-1);
                % -- FoT ---------------------
                if (ky(i+1,j)/ky(i,j)) > 1.1 || (ky(i+1,j)/ky(i,j)) < 0.9 %detect change in material
                    FoT = (ky(i,j)*(delT/2)+ky(i+1,j)*(delT/2))*DT/(rho(i,j)*Cp(i,j)*delT*delT*delT);
                end
                % -- FoL -------------------------
                if (kx(i,j-1)/kx(i,j)) > 1.1 || (kx(i,j-1)/kx(i,j)) < 0.9 %detect change in material
                    FoL = (kx(i,j)*(delL/2)+kx(i,j-1)*(delL/2))*DT/(rho(i,j)*Cp(i,j)*delL*delL*delL);
                end
                
                %simplification variables
                b = 0.5*FoB + 0.5*FoT*BiB + 0.5*FoT*BiRadB + 0.5*FosB ...
                  + 0.5*FoT + 0.5*FoB*BiT + 0.5*FoB*BiRadT + 0.5*FosT ...
                  + 0.5*FoL + 0.5*FoR*BiL + 0.5*FoR*BiRadL + 0.5*FosL ...
                  + 0.5*FoR + 0.5*FoL*BiR + 0.5*FoL*BiRadR + 0.5*FosR;
                c = -0.5*FoT;
                d = -0.5*FoL;
                f = 0;
                BCs = FosB*TsB(j) + FoT*BiB*TfB(j) + FoT*BiRadB*TrB(j) ...
                    + FosR*TsR(i) + FoL*BiR*TfR(i) + FoL*BiRadR*TrR(i);
                
                %assign vector values
                B(indB) = 1+b;
                C(indC) = c;
                D(indD) = d;
                F(indF) = f;
                z(indz) = (1-b)*To(i,j) - c*To(i+1,j) - d*To(i,j-1) + BCs;
                
                %update indices
                indB = indB + 1;
                indC = indC + 1;
                indD = indD + 1;
                indF = indF + 1;
                indz = indz + 1;
                
            %BOTTOM NON-CORNER NODE
            else
                
                %Fouier numbers and Biot numbers, etc.
                %bottom vars
                FoB = 0;
                BiB = hB(j)*AB(j)*JBy(j)/ky(i,j); %Boit number
                BiRadB = uB(j)*AB(j)*JBy(j)/ky(i,j); %analogous Boit number for radiation
                FosB = DT*CB(j)/(rho(i,j)*Cp(i,j)*VB(j));
                %top vars
                FoT = DT*ky(i,j)*(1/JBy(j))/(rho(i,j)*Cp(i,j)*VB(j)); %Fourier number;
                BiT = 0;
                BiRadT = 0;
                FosT = 0;
                %left vars
                FoL = DT*kx(i,j)*(1/JBx(j-1))/(rho(i,j)*Cp(i,j)*VB(j));
                BiL = 0;
                BiRadL = 0;
                FosL = 0;
                %right vars
                FoR = DT*kx(i,j)*(1/JBx(j))/(rho(i,j)*Cp(i,j)*VB(j));
                BiR = 0;
                BiRadR = 0;
                FosR = 0;
                
                %adjust Fourier numbers for material transiton
                delT = y(i+1) - y(i);
                delL = x(j) - x(j-1);
                delR = x(j+1) - x(j);
                % -- FoT ---------------------
                if (ky(i+1,j)/ky(i,j)) > 1.1 || (ky(i+1,j)/ky(i,j)) < 0.9 %detect change in material
                    FoT = (ky(i,j)*(delT/2)+ky(i+1,j)*(delT/2))*DT/(rho(i,j)*Cp(i,j)*delT*delT*delT);
                end
                % -- FoL -------------------------
                if (kx(i,j-1)/kx(i,j)) > 1.1 || (kx(i,j-1)/kx(i,j)) < 0.9 %detect change in material
                    FoL = (kx(i,j)*(delL/2)+kx(i,j-1)*(delL/2))*DT/(rho(i,j)*Cp(i,j)*delL*delL*delL);
                end
                % -- FoR -------------------------
                if (kx(i,j+1)/kx(i,j)) > 1.1 || (kx(i,j+1)/kx(i,j)) < 0.9 %detect change in material
                    FoR = (kx(i,j)*(delR/2)+kx(i,j+1)*(delR/2))*DT/(rho(i,j)*Cp(i,j)*delR*delR*delR);
                end
                  
                %simplification variables
                b = 0.5*FoB + 0.5*FoT*BiB + 0.5*FoT*BiRadB + 0.5*FosB ...
                  + 0.5*FoT + 0.5*FoB*BiT + 0.5*FoB*BiRadT + 0.5*FosT ...
                  + 0.5*FoL + 0.5*FoR*BiL + 0.5*FoR*BiRadL + 0.5*FosL ...
                  + 0.5*FoR + 0.5*FoL*BiR + 0.5*FoL*BiRadR + 0.5*FosR;
                c = -0.5*FoT;
                d = -0.5*FoL;
                f = -0.5*FoR;
                BCs = FosB*TsB(j) + FoT*BiB*TfB(j) + FoT*BiRadB*TrB(j);
                
                %assign vector values
                B(indB) = 1+b;
                C(indC) = c;
                D(indD) = d;
                F(indF) = f;
                z(indz) = (1-b)*To(i,j) - c*To(i+1,j) - d*To(i,j-1) - f*To(i,j+1) + BCs;
                
                %update indices
                indB = indB + 1;
                indC = indC + 1;
                indD = indD + 1;
                indF = indF + 1;
                indz = indz + 1;
                
            end
        
        %TOP SURFACE
        elseif i == m
            
            %TOP LEFT CORNER NODE
            if j == 1
                
                %Fourier numbers and Boit numbers, etc.
                %left vars
                FoL = 0;
                BiL = hL(i)*AL(i)*JLx(i)/kx(i,j); %Boit number
                BiRadL = uL(i)*AL(i)*JLx(i)/kx(i,j); %analogous Boit number for radiation
                FosL = DT*CL(i)/(rho(i,j)*Cp(i,j)*VL(i));
                %right vars 
                FoR = DT*kx(i,j)*(1/JLx(i))/(rho(i,j)*Cp(i,j)*VL(i)); %Fourier number;
                BiR = 0;
                BiRadR = 0;
                FosR = 0;
                %bottom vars
                FoB = DT*ky(i,j)*(1/JTy(j))/(rho(i,j)*Cp(i,j)*VT(j)); %Fourier number;
                BiB = 0;
                BiRadB = 0;
                FosB = 0;
                %top vars
                FoT = 0;
                BiT = hT(j)*AT(j)*JTy(j)/ky(i,j); %Boit number
                BiRadT = uT(j)*AT(j)*JTy(j)/ky(i,j); %analogous Boit number for radiation
                FosT = DT*CT(j)/(rho(i,j)*Cp(i,j)*VT(j));
                
                %adjust Fourier numbers for material transiton
                delB = y(i) - y(i-1);
                delR = x(j+1) - x(j);
                % -- FoB ---------------------
                if (ky(i-1,j)/ky(i,j)) > 1.1 || (ky(i-1,j)/ky(i,j)) < 0.9 %detect change in material
                    FoB = (ky(i,j)*(delB/2)+ky(i-1,j)*(delB/2))*DT/(rho(i,j)*Cp(i,j)*delB*delB*delB);
                end
                % -- FoR -------------------------
                if (kx(i,j+1)/kx(i,j)) > 1.1 || (kx(i,j+1)/kx(i,j)) < 0.9 %detect change in material
                    FoR = (kx(i,j)*(delR/2)+kx(i,j+1)*(delR/2))*DT/(rho(i,j)*Cp(i,j)*delR*delR*delR);
                end
                
                %simplification variables
                b = 0.5*FoB + 0.5*FoT*BiB + 0.5*FoT*BiRadB + 0.5*FosB ...
                  + 0.5*FoT + 0.5*FoB*BiT + 0.5*FoB*BiRadT + 0.5*FosT ...
                  + 0.5*FoL + 0.5*FoR*BiL + 0.5*FoR*BiRadL + 0.5*FosL ...
                  + 0.5*FoR + 0.5*FoL*BiR + 0.5*FoL*BiRadR + 0.5*FosR;
                g = -0.5*FoB;
                d = 0;
                f = -0.5*FoR;
                BCs = FosT*TsT(j) + FoB*BiT*TfT(j) + FoB*BiRadT*TrT(j) ...
                    + FosL*TsL(i) + FoR*BiL*TfL(i) + FoR*BiRadL*TrL(i);
                
                %assign vector values
                G(indG) = g;
                B(indB) = 1+b;
                D(indD) = d;
                F(indF) = f;
                z(indz) = -g*To(i-1,j) + (1-b)*To(i,j) - f*To(i,j+1) + BCs;
                
                %update indices
                indG = indG + 1;
                indB = indB + 1;
                indD = indD + 1;
                indF = indF + 1;
                indz = indz + 1;
                
            %TOP RIGHT CORNER NODE
            elseif j == n
                
                %Fouier number and Biot Numbers, etc.
                %left vars
                FoL = DT*kx(i,j)*(1/JRx(i))/(rho(i,j)*Cp(i,j)*VR(i)); %Fourier number;
                BiL = 0;
                BiRadL = 0;
                FosL = 0;
                %right vars (conduction)
                FoR = 0;
                BiR = hR(i)*AR(i)*JRx(i)/kx(i,j); %Boit number
                BiRadR = uR(i)*AR(i)*JRx(i)/kx(i,j); %analogous Boit number for radiation
                FosR = DT*CR(i)/(rho(i,j)*Cp(i,j)*VR(i));
                %bottom vars
                FoB = DT*ky(i,j)*(1/JTy(j))/(rho(i,j)*Cp(i,j)*VT(j)); %Fourier number;
                BiB = 0;
                BiRadB = 0;
                FosB = 0;
                %top bars
                FoT = 0;
                BiT = hT(j)*AT(j)*JTy(j)/ky(i,j); %Boit number
                BiRadT = uT(j)*AT(j)*JTy(j)/ky(i,j); %analogous Boit number for radiation
                FosT = DT*CT(j)/(rho(i,j)*Cp(i,j)*VT(j));
                
                %adjust Fourier numbers for material transiton
                delB = y(i) - y(i-1);
                delL = x(j) - x(j-1);
                % -- FoB ---------------------
                if (ky(i-1,j)/ky(i,j)) > 1.1 || (ky(i-1,j)/ky(i,j)) < 0.9 %detect change in material
                    FoB = (ky(i,j)*(delB/2)+ky(i-1,j)*(delB/2))*DT/(rho(i,j)*Cp(i,j)*delB*delB*delB);
                end
                % -- FoL -------------------------
                if (kx(i,j-1)/kx(i,j)) > 1.1 || (kx(i,j-1)/kx(i,j)) < 0.9 %detect change in material
                    FoL = (kx(i,j)*(delL/2)+kx(i,j-1)*(delL/2))*DT/(rho(i,j)*Cp(i,j)*delL*delL*delL);
                end
                
                %simplification variables
                b = 0.5*FoB + 0.5*FoT*BiB + 0.5*FoT*BiRadB + 0.5*FosB ...
                  + 0.5*FoT + 0.5*FoB*BiT + 0.5*FoB*BiRadT + 0.5*FosT ...
                  + 0.5*FoL + 0.5*FoR*BiL + 0.5*FoR*BiRadL + 0.5*FosL ...
                  + 0.5*FoR + 0.5*FoL*BiR + 0.5*FoL*BiRadR + 0.5*FosR;
                g = -0.5*FoB;
                d = -0.5*FoL;
                BCs = FosT*TsT(j) + FoB*BiT*TfT(j) + FoB*BiRadT*TrT(j) ...
                    + FosR*TsR(i) + FoL*BiR*TfR(i) + FoL*BiRadR*TrR(i);
                
                %assign vector values
                G(indG) = g;
                B(indB) = 1+b;
                D(indD) = d;
                z(indz) = -g*To(i-1,j) + (1-b)*To(i,j) - d*To(i,j-1) + BCs;
                
                %update indices
                indG = indG + 1;
                indB = indB + 1;
                indD = indD + 1;
                indz = indz + 1;
                
            %TOP NON-CORNER NODE
            else
                
                %Fouier numbers and Biot numbers, etc.
                FoB = DT*ky(i,j)*(1/JTy(j))/(rho(i,j)*Cp(i,j)*VT(j)); %Fourier number;
                BiB = 0;
                BiRadB = 0;
                FosB = 0;
                %top vars
                FoT = 0;
                BiT = hT(j)*AT(j)*JTy(j)/ky(i,j); %Boit number
                BiRadT = uT(j)*AT(j)*JTy(j)/ky(i,j); %analogous Boit number for radiation
                FosT = DT*CT(j)/(rho(i,j)*Cp(i,j)*VT(j));
                %left vars
                FoL = DT*kx(i,j)*(1/JTx(j-1))/(rho(i,j)*Cp(i,j)*VT(j));
                BiL = 0;
                BiRadL = 0;
                FosL = 0;
                %right vars
                FoR = DT*kx(i,j)*(1/JTx(j))/(rho(i,j)*Cp(i,j)*VT(j));
                BiR = 0;
                BiRadR = 0;
                FosR = 0;
                
                %adjust Fourier numbers for material transiton
                delB = y(i) - y(i-1);
                delL = x(j) - x(j-1);
                delR = x(j+1) - x(j);
                % -- FoB ---------------------
                if (ky(i-1,j)/ky(i,j)) > 1.1 || (ky(i-1,j)/ky(i,j)) < 0.9 %detect change in material
                    FoB = (ky(i,j)*(delB/2)+ky(i-1,j)*(delB/2))*DT/(rho(i,j)*Cp(i,j)*delB*delB*delB);
                end
                % -- FoL -------------------------
                if (kx(i,j-1)/kx(i,j)) > 1.1 || (kx(i,j-1)/kx(i,j)) < 0.9 %detect change in material
                    FoL = (kx(i,j)*(delL/2)+kx(i,j-1)*(delL/2))*DT/(rho(i,j)*Cp(i,j)*delL*delL*delL);
                end
                % -- FoR -------------------------
                if (kx(i,j+1)/kx(i,j)) > 1.1 || (kx(i,j+1)/kx(i,j)) < 0.9 %detect change in material
                    FoR = (kx(i,j)*(delR/2)+kx(i,j+1)*(delR/2))*DT/(rho(i,j)*Cp(i,j)*delR*delR*delR);
                end
                
                %simplification variables
                b = 0.5*FoB + 0.5*FoT*BiB + 0.5*FoT*BiRadB + 0.5*FosB ...
                  + 0.5*FoT + 0.5*FoB*BiT + 0.5*FoB*BiRadT + 0.5*FosT ...
                  + 0.5*FoL + 0.5*FoR*BiL + 0.5*FoR*BiRadL + 0.5*FosL ...
                  + 0.5*FoR + 0.5*FoL*BiR + 0.5*FoL*BiRadR + 0.5*FosR;
                g = -0.5*FoB;
                d = -0.5*FoL;
                f = -0.5*FoR;
                BCs = FosT*TsT(j) + FoB*BiT*TfT(j) + FoB*BiRadT*TrT(j);
                
                %assign vector values
                G(indG) = g;
                B(indB) = 1+b;
                D(indD) = d;
                F(indF) = f;
                z(indz) = -g*To(i-1,j) + (1-b)*To(i,j) - d*To(i,j-1) - f*To(i,j+1) + BCs;
                
                %update indices
                indG = indG + 1;
                indB = indB + 1;
                indD = indD + 1;
                indF = indF + 1;
                indz = indz + 1;
                
            end
            
        %ROW IS BETWEEN THE TOP AND BOTTOM SURFACES
        else
            
            %LEFT SURFACE NON-CORNER NODE
            if j == 1
                
                %Fourier numbers and Boit numbers
                %left vars
                FoL = 0;
                BiL = hL(i)*AL(i)*JLx(i)/kx(i,j); %Boit number
                BiRadL = uL(i)*AL(i)*JLx(i)/kx(i,j); %analogous Boit number for radiation
                FosL = DT*CL(i)/(rho(i,j)*Cp(i,j)*VL(i));
                %right vars 
                FoR = DT*kx(i,j)*(1/JLx(i))/(rho(i,j)*Cp(i,j)*VL(i)); %Fourier number;
                BiR = 0;
                BiRadR = 0;
                FosR = 0;
                %bottom vars
                FoB = DT*ky(i,j)*(1/JLy(i-1))/(rho(i,j)*Cp(i,j)*VL(i));
                BiB = 0;
                BiRadB = 0;
                FosB = 0;
                %top vars
                FoT = DT*ky(i,j)*(1/JLy(i))/(rho(i,j)*Cp(i,j)*VL(i));
                BiT = 0;
                BiRadT = 0;
                FosT = 0;
                
                %adjust Fourier numbers for material transiton
                delB = y(i) - y(i-1);
                delT = y(i+1) - y(i);
                delR = x(j+1) - x(j);
                % -- FoB ---------------------
                if (ky(i-1,j)/ky(i,j)) > 1.1 || (ky(i-1,j)/ky(i,j)) < 0.9 %detect change in material
                    FoB = (ky(i,j)*(delB/2)+ky(i-1,j)*(delB/2))*DT/(rho(i,j)*Cp(i,j)*delB*delB*delB);
                end
                % -- FoT ---------------------
                if (ky(i+1,j)/ky(i,j)) > 1.1 || (ky(i+1,j)/ky(i,j)) < 0.9 %detect change in material
                    FoT = (ky(i,j)*(delT/2)+ky(i+1,j)*(delT/2))*DT/(rho(i,j)*Cp(i,j)*delT*delT*delT);
                end
                % -- FoR -------------------------
                if (kx(i,j+1)/kx(i,j)) > 1.1 || (kx(i,j+1)/kx(i,j)) < 0.9 %detect change in material
                    FoR = (kx(i,j)*(delR/2)+kx(i,j+1)*(delR/2))*DT/(rho(i,j)*Cp(i,j)*delR*delR*delR);
                end
                
                %simplification variables
                b = 0.5*FoB + 0.5*FoT*BiB + 0.5*FoT*BiRadB + 0.5*FosB ...
                  + 0.5*FoT + 0.5*FoB*BiT + 0.5*FoB*BiRadT + 0.5*FosT ...
                  + 0.5*FoL + 0.5*FoR*BiL + 0.5*FoR*BiRadL + 0.5*FosL ...
                  + 0.5*FoR + 0.5*FoL*BiR + 0.5*FoL*BiRadR + 0.5*FosR;
                g = -0.5*FoB;
                c = -0.5*FoT;
                d = 0;
                f = -0.5*FoR;
                BCs = FosL*TsL(i) + FoR*BiL*TfL(i) + FoR*BiRadL*TrL(i);
                
                %assign vector values
                G(indG) = g;
                B(indB) = 1+b;
                C(indC) = c;
                D(indD) = d;
                F(indF) = f;
                z(indz) = -g*To(i-1,j) + (1-b)*To(i,j) - c*To(i+1,j) - f*To(i,j+1) + BCs;
                
                %update indices
                indG = indG + 1;
                indB = indB + 1;
                indC = indC + 1;
                indD = indD + 1;
                indF = indF + 1;
                indz = indz + 1;
                
            %RIGHT SURFACE NON-CORNER NODE
            elseif j == n
                
                %Fourier numbers and Boit numbers
                %bottom vars
                FoB = DT*ky(i,j)*(1/JRy(i-1))/(rho(i,j)*Cp(i,j)*VR(i)); %Fourier number;
                BiB = 0; %Boit number
                BiRadB = 0; %analogous Boit number for radiation
                FosB = 0;
                %top vars
                FoT = DT*ky(i,j)*(1/JRy(i))/(rho(i,j)*Cp(i,j)*VR(i)); %Fourier number;
                BiT = 0;
                BiRadT = 0;
                FosT = 0;
                %left vars
                FoL = DT*kx(i,j)*(1/JRx(i))/(rho(i,j)*Cp(i,j)*VR(i)); %Fourier number;
                BiL = 0;
                BiRadL = 0;
                FosL = 0;
                %right vars
                FoR = 0;
                BiR = hR(i)*AR(i)*JRx(i)/kx(i,j); %Boit number
                BiRadR = uR(i)*AR(i)*JRx(i)/kx(i,j); %analogous Boit number for radiation
                FosR = DT*CR(i)/(rho(i,j)*Cp(i,j)*VR(i));
                
                %adjust Fourier numbers for material transiton
                delB = y(i) - y(i-1);
                delT = y(i+1) - y(i);
                delL = x(j) - x(j-1);
                % -- FoB ---------------------
                if (ky(i-1,j)/ky(i,j)) > 1.1 || (ky(i-1,j)/ky(i,j)) < 0.9 %detect change in material
                    FoB = (ky(i,j)*(delB/2)+ky(i-1,j)*(delB/2))*DT/(rho(i,j)*Cp(i,j)*delB*delB*delB);
                end
                % -- FoT ---------------------
                if (ky(i+1,j)/ky(i,j)) > 1.1 || (ky(i+1,j)/ky(i,j)) < 0.9 %detect change in material
                    FoT = (ky(i,j)*(delT/2)+ky(i+1,j)*(delT/2))*DT/(rho(i,j)*Cp(i,j)*delT*delT*delT);
                end
                % -- FoL -------------------------
                if (kx(i,j-1)/kx(i,j)) > 1.1 || (kx(i,j-1)/kx(i,j)) < 0.9 %detect change in material
                    FoL = (kx(i,j)*(delL/2)+kx(i,j-1)*(delL/2))*DT/(rho(i,j)*Cp(i,j)*delL*delL*delL);
                end
                
                %simplification variables
                b = 0.5*FoB + 0.5*FoT*BiB + 0.5*FoT*BiRadB + 0.5*FosB ...
                  + 0.5*FoT + 0.5*FoB*BiT + 0.5*FoB*BiRadT + 0.5*FosT ...
                  + 0.5*FoL + 0.5*FoR*BiL + 0.5*FoR*BiRadL + 0.5*FosL ...
                  + 0.5*FoR + 0.5*FoL*BiR + 0.5*FoL*BiRadR + 0.5*FosR;
                g = -0.5*FoB;
                c = -0.5*FoT;
                d = -0.5*FoL;
                f = 0;
                BCs = FosR*TsR(i) + FoL*BiR*TfR(i) + FoL*BiRadR*TrR(i);
                
                %assign vector values
                G(indG) = g;
                B(indB) = 1+b;
                C(indC) = c;
                D(indD) = d;
                F(indF) = f;
                z(indz) = -g*To(i-1,j) + (1-b)*To(i,j) - c*To(i+1,j) - d*To(i,j-1) + BCs;
                
                %update indices
                indG = indG + 1;
                indB = indB + 1;
                indC = indC + 1;
                indD = indD + 1;
                indF = indF + 1;
                indz = indz + 1;
                
            %INTERIOR NODE
            else
                
                %Fourier and Biot numbers, etc.
                % distance between nodes
                del1 = y(i) - y(i-1);
                del2 = y(i+1) - y(i);
                del3 = x(j) - x(j-1);
                del4 = x(j+1) - x(j);
                % simplification coefficients (for spatial discretization)
                C3 = 1 + (del1^3/del2^2 - del1)/(del2 + del1);
                C2 = 1 + (del1/del2)^3;
                C1 = (del1/del2)^3 - ((del1^3/del2^2) - del1)/(del2+del1);
                C6 = 1 + (del3^3/del4^2 - del3)/(del4 + del3);
                C5 = 1 + (del3/del4)^3;
                C4 = (del3/del4)^3 - ((del3^3/del4^2) - del3)/(del4+del3);
                % calculated Fourier numbers
                Fo_y = 2*ky(i,j)*DT/(rho(i,j)*Cp(i,j)*(del1^2 + del1^3/del2)); %Fourier number
                Fok_y = (DT/(rho(i,j)*Cp(i,j)*(del1+del2)))*((ky(i+1,j)-ky(i-1,j))/(del1+del2) + ky(i,j)*a/y(i)); %Fourier number for conductivity variation and shape
                Fo_x = 2*kx(i,j)*DT/(rho(i,j)*Cp(i,j)*(del3^2 + del3^3/del4)); %Fourier number
                Fok_x = (DT/(rho(i,j)*Cp(i,j)*(del3+del4)))*((kx(i,j+1)-kx(i,j-1))/(del3+del4) + kx(i,j)*q/x(j)); %Fourier number for conductivity variation and shape
                % adjust equations for change in materials
                %   when there is a change in materials the transition in materials
                %   properties, most notabely thermal conductivity, is abrupt. This
                %   discontinuty can cause accuracy and stability issues with the 
                %   derivative term dk/dt = (k(i+1)-k(i-1))/(del1+del2). Therefore a
                %   more robust approach is utilized when a material transition is
                %   detected. This method is document in "Integrated Turbine Tip
                %   Clearance and Gas Turbine Engine Simulation" by J. Chapman, J.
                %   Kratz, T.-H. Guo, and J. Litt. The method uses a transition Fourier
                %   number to address the discontinuity. The method from this reference
                %   has been generalized for non-uniform discretizations and geometries
                %   that could be either planar or cylindrical. When there is not a
                %   transition in materials the dk/dt term should be better
                %   approximated with the central difference scheme that is used and
                %   the standard formulation will be utilized. Material transition is
                %   detected by a sigificant (10%) increase or decrease in thermal 
                %   conductivity.
                % -- y-dir ---------------------
                if (ky(i+1,j)/ky(i,j)) > 1.1 || (ky(i+1,j)/ky(i,j)) < 0.9 %detect change in material
                    Fo_y = ky(i,j)*DT/(rho(i,j)*Cp(i,j)*del1^2);
                    Fok_y = (DT/(rho(i,j)*Cp(i,j)*(del1+del2)))*ky(i,j)*a/y(i);
                    Fob_y = (ky(i,j)*(del2/2)+ky(i+1,j)*(del2/2))*DT/(rho(i,j)*Cp(i,j)*del2*del1*del2);
                    K1 = Fo_y;
                    K2 = 2*0.5*(Fo_y+Fob_y); 
                    K3 = Fob_y;
                elseif (ky(i,j)/ky(i-1,j)) > 1.1 || (ky(i,j)/ky(i-1,j)) < 0.9 %detect change in material
                    Fo_y = ky(i,j)*DT/(rho(i,j)*Cp(i,j)*del2^2);
                    Fok_y = (DT/(rho(i,j)*Cp(i,j)*(del1+del2)))*ky(i,j)*a/y(i);
                    Foa_y = (ky(i,j)*(del1/2)+ky(i-1,j)*(del1/2))*DT/(rho(i,j)*Cp(i,j)*del1*del1*del2);
                    K1 = Foa_y;
                    K2 = 2*0.5*(Fo_y+Foa_y); 
                    K3 = Fo_y;
                else % no change in material detected - go with standard solution
                    K1 = C1*Fo_y;
                    K2 = C2*Fo_y;
                    K3 = C3*Fo_y;
                end
                % -- x-dir -------------------------
                if (kx(i,j+1)/kx(i,j)) > 1.1 || (kx(i,j+1)/kx(i,j)) < 0.9 %detect change in material
                    Fo_x = kx(i,j)*DT/(rho(i,j)*Cp(i,j)*del3^2);
                    Fok_x = (DT/(rho(i,j)*Cp(i,j)*(del3+del4)))*kx(i,j)*q/x(j);
                    Fob_x = (kx(i,j)*(del4/2)+kx(i,j+1)*(del4/2))*DT/(rho(i,j)*Cp(i,j)*del4*del3*del4);
                    K4 = Fo_x;
                    K5 = 2*0.5*(Fo_x+Fob_x); 
                    K6 = Fob_x;
                elseif (kx(i,j)/kx(i,j-1)) > 1.1 || (kx(i,j)/kx(i,j-1)) < 0.9 %detect change in material
                    Fo_x = kx(i,j)*DT/(rho(i,j)*Cp(i,j)*del4^2);
                    Fok_x = (DT/(rho(i,j)*Cp(i,j)*(del3+del4)))*kx(i,j)*q/x(j);
                    Foa_x = (kx(i,j)*(del3/2)+kx(i,j-1)*(del3/2))*DT/(rho(i,j)*Cp(i,j)*del3*del3*del4);
                    K4 = Foa_x;
                    K5 = 2*0.5*(Fo_x+Foa_x); 
                    K6 = Fo_x;
                else % no change in material detected - go with standard solution
                    K4 = C4*Fo_x;
                    K5 = C5*Fo_x;
                    K6 = C6*Fo_x;
                end
                
                %simplification variables
                g = 0.5*Fok_y - 0.5*K1;
                b = 0.5*K2 + 0.5*K5;
                c = -0.5*Fok_y - 0.5*K3;
                d = 0.5*Fok_x - 0.5*K4;
                f = -0.5*Fok_x - 0.5*K6;
                
                %assign vector values
                G(indG) = g;
                B(indB) = 1+b;
                C(indC) = c;
                D(indD) = d;
                F(indF) = f;
                z(indz) = -g*To(i-1,j) + (1-b)*To(i,j) - c*To(i+1,j) - d*To(i,j-1) - f*To(i,j+1);
                
                %update indices
                indG = indG + 1;
                indB = indB + 1;
                indC = indC + 1;
                indD = indD + 1;
                indF = indF + 1;
                indz = indz + 1;
                
            end
            
        end
    
    end
    
end

    
% Build matrix A ---------------------------------------------------------%

% Modify with B 
for ii = 1:length(B)
    A(ii,ii) = B(ii);
end

% Modify with D
for ii = 1:length(D)
    A(ii+1,ii) = D(ii);
end

% Modify with F
for ii = 1:length(F)
    A(ii,ii+1) = F(ii);
end

% Modify with C
for ii = 1:length(C)
    A(ii,ii+n) = C(ii);
end

% Modify with G 
for ii = 1:length(G)
    A(ii+n,ii) = G(ii);
end

% Solve the system of equations ------------------------------------------%

Tvec = A\z;

% Convert to Matrix form -------------------------------------------------%

T = zeros(m,n);
for i = 1:m
    for j = 1:n
        T(i,j) = Tvec((i-1)*n+j);
    end
end

Z = zeros(m,n);
for i = 1:m
    for j = 1:n
        Z(i,j) = z((i-1)*n+j);
    end
end

% END OF CODE ------------------------------------------------------------%
